simulink subsystem "control_law"  (R2023a)
settings: Solver=VariableStepAuto  StartTime=0.0  StopTime=10.0  RelTol=1e-3
values from neighbouring files (symbols this model uses):
  Kp_x = K(:,3:5)    [LQR_PI.m]    (also in full_loop.m = K(:,nref+1:np+nref); inner_loop.m = K(:,4:9))
undefined symbols (not defined in the file or in its folder): Kp_p, Kp_pitch, Kp_q, Kp_r, Kp_roll, Kp_vx, Kp_vy, Kp_vz, Kp_y, Kp_yaw, Kp_z, param, sat_p, sat_pitch, sat_q, sat_r, sat_roll, sat_Vx, sat_Vy, sat_Vz, sat_yaw, Td, Td_pos, Ti, Ti_pos
libraries: slpidlib x4, dspfdesign x3
settings Model: Creator=timme  LastModifiedBy=timme

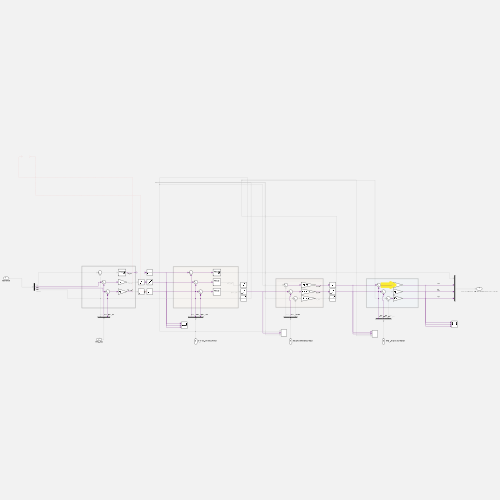
[thumbnail: Simulink's stored preview of the top-level diagram]
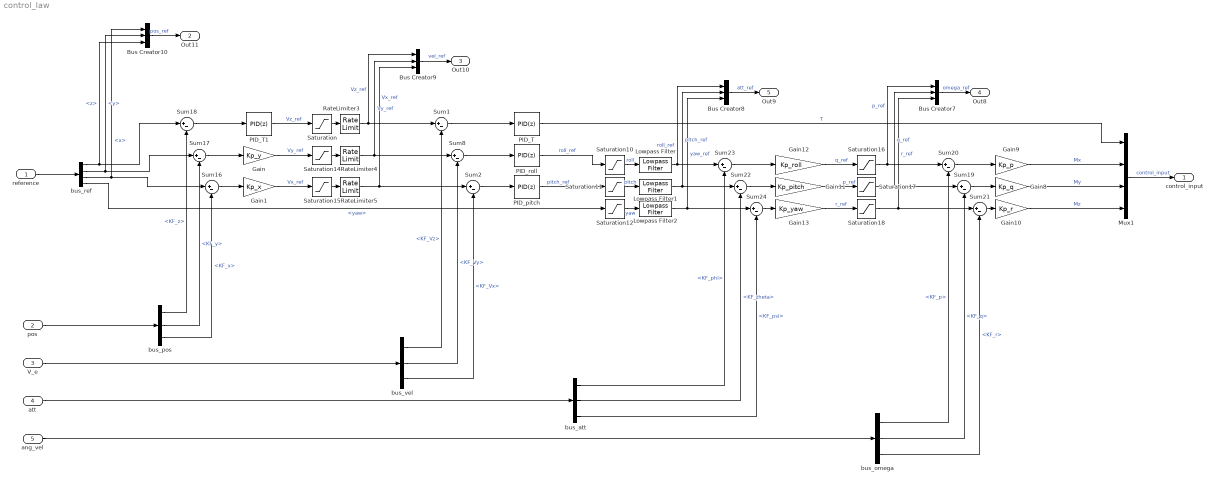
== system control_law ==
  reference : Inport
  pos : Inport  Port=2  Unit=m
  V_e : Inport  Port=3  Unit=m/s
  att : Inport  Port=4  Unit=rad
  ang_vel : Inport  Port=5  Unit=rad/s
  Bus Creator{7..10} (4 alike) : BusCreator  Inputs=3
  Gain : Gain  Gain=Kp_y
  Gain1 : Gain  Gain=Kp_x
  Gain10 : Gain  Gain=Kp_r
  Gain11 : Gain  Gain=Kp_pitch
  Gain12 : Gain  Gain=Kp_roll
  Gain13 : Gain  Gain=Kp_yaw
  Gain8 : Gain  Gain=Kp_q
  Gain9 : Gain  Gain=Kp_p
  Lowpass Filter : dspfdesign/Lowpass Filter  FilterType=IIR  DesignForMinimumOrder=on  FilterOrder=50  PassbandFrequency=1  StopbandFrequency=100  PassbandRipple=0.1  StopbandAttenuation=50  SampleRateMode=Specify on dialog  SampleRate=1000  SimulateUsing=Interpreted execution  roundingMode=Floor  coeffsDataTypeStr=fixdt(1,16)
  Lowpass Filter1 : dspfdesign/Lowpass Filter  FilterType=IIR  DesignForMinimumOrder=on  FilterOrder=50  PassbandFrequency=1  StopbandFrequency=100  PassbandRipple=0.1  StopbandAttenuation=50  SampleRateMode=Specify on dialog  SampleRate=1000  SimulateUsing=Interpreted execution  roundingMode=Floor  coeffsDataTypeStr=fixdt(1,16)
  Lowpass Filter2 : dspfdesign/Lowpass Filter  FilterType=IIR  DesignForMinimumOrder=on  FilterOrder=50  PassbandFrequency=1  StopbandFrequency=100  PassbandRipple=0.1  StopbandAttenuation=50  SampleRateMode=Specify on dialog  SampleRate=1000  SimulateUsing=Interpreted execution  roundingMode=Floor  coeffsDataTypeStr=fixdt(1,16)
  Mux1 : Mux
  PID_T : slpidlib/PID Controller  Controller=PID  Form=Parallel  TimeDomain=Discrete-time  UseExternalTs=off  SampleTime=param.dt  IntegratorMethod=Forward Euler  FilterMethod=Forward Euler  ControllerParametersSource=internal  P=Kp_vz  I=0  UseKiTs=on  D=0  N=100  UseFilter=on  TunerSelectOption=Transfer Function Based (PID Tuner App)  InitialConditionSource=internal  InitialConditionForIntegrator=0  InitialConditionForFilter=0  DifferentiatorICPrevScaledInput=0  ExternalReset=none  TrackingMode=off  Kt=1  LimitOutput=on  SatLimitsSource=internal  UpperSaturationLimit=2*param.m*param.g  LowerSaturationLimit=-2*param.m*param.g  LinearizeAsGain=on  AntiWindupMode=back-calculation  Kb=1  LimitIntegrator=off  UpperIntegratorSaturationLimit=inf  LowerIntegratorSaturationLimit=-inf  POutMin=[]  POutMax=[]  IOutMin=[]  IOutMax=[]  DOutMin=[]  DOutMax=[]  NOutMin=[]  NOutMax=[]  SumOutMin=[]  SumOutMax=[]  SaturationOutMin=[]  SaturationOutMax=[]  PParamMin=[]  PParamMax=[]  IParamMin=[]  IParamMax=[]  DParamMin=[]  DParamMax=[]  NParamMin=[]  NParamMax=[]  KbParamMin=[]  KbParamMax=[]  KtParamMin=[]  KtParamMax=[]  KbOutMin=[]  KbOutMax=[]  KtOutMin=[]  KtOutMax=[]  IntegratorOutMin=[]  IntegratorOutMax=[]  FilterOutMin=[]  FilterOutMax=[]  SumI1OutMin=[]  SumI1OutMax=[]  SumI2OutMin=[]  SumI2OutMax=[]  SumI3OutMin=[]  SumI3OutMax=[]  SumI4OutMin=[]  SumI4OutMax=[]  SumDOutMin=[]  SumDOutMax=[]  DifferentiatorOutMin=[]  DifferentiatorOutMax=[]  FilterDiffOutCoefMin=[]  FilterDiffOutCoefMax=[]  ReciprocalOutMin=[]  ReciprocalOutMax=[]  SumDenOutMin=[]  SumDenOutMax=[]  SumNumOutMin=[]  SumNumOutMax=[]  DivideOutMin=[]  DivideOutMax=[]  UdiffTsProdOutMin=[]  UdiffTsProdOutMax=[]  NTsProdOutMin=[]  NTsProdOutMax=[]  UintegralTsProdOutMin=[]  UintegralTsProdOutMax=[]  UngainTsProdOutMin=[]  UngainTsProdOutMax=[]  ClampingZeroOutDataTypeStr=Inherit: Inherit via back propagation  ClampingZeroOutMin=[]  ClampingZeroOutMax=[]  FilterDenConstantOutDataTypeStr=Inherit: Inherit via back propagation  FilterDenConstantOutMin=[]  FilterDenConstantOutMax=[]  PCopyOutDataTypeStr=Inherit: Inherit via back propagation  PCopyOutMin=[]  PCopyOutMax=[]  NCopyOutDataTypeStr=Inherit: Inherit via back propagation  NCopyOutMin=[]  NCopyOutMax=[]  IntegratorContinuousStateAttributes=''  IntegratorStateMustResolveToSignalObject=off  IntegratorRTWStateStorageClass=Auto  FilterContinuousStateAttributes=''  FilterStateMustResolveToSignalObject=off  FilterRTWStateStorageClass=Auto  ParallelPVariant=InternalParameters  IdealPVariant=Disabled  IVariant=InternalParameters  DVariant=InternalParameters  IntegratorVariant=Discrete  SatVariant=Enabled  AWVariant=BackCalculation  PCopyVariant=Disabled  TRVariant=Disabled  FdbkBlocksVariant=Forward  IdealPFdbkVariant=Disabled  SatFdbkVariant=Disabled  DerivativeFilterVariant=ForwardEulerFilter  NVariant=InternalParameters  NCopyVariant=Disabled  FilterICVariant=InternalICsFilter  IntegratorICVariant=InternalICs  ExternalResetVariant=Disabled  TRSumVariant=Passthrough  SumFdbkVariant=Disabled  SumVariant=Sum_PID  TsampFilterVariant=InternalTs  TsampNgainVariant=Passthrough  TsampIntegralVariant=Disabled_SignalSpec  ExternalSaturationOutDataTypeStr=Inherit: Same as second input
  PID_T1 : slpidlib/PID Controller  Controller=PID  Form=Parallel  TimeDomain=Discrete-time  UseExternalTs=off  SampleTime=param.dt  IntegratorMethod=Forward Euler  FilterMethod=Forward Euler  ControllerParametersSource=internal  P=Kp_z*(1+Td_pos/Ti_pos)  I=Kp_z/Ti_pos*param.dt  UseKiTs=on  D=Kp_z*Td_pos  N=100  UseFilter=on  TunerSelectOption=Transfer Function Based (PID Tuner App)  InitialConditionSource=internal  InitialConditionForIntegrator=0  InitialConditionForFilter=0  DifferentiatorICPrevScaledInput=0  ExternalReset=none  TrackingMode=off  Kt=1  LimitOutput=on  SatLimitsSource=internal  UpperSaturationLimit=sat_Vz  LowerSaturationLimit=-sat_Vz  LinearizeAsGain=on  AntiWindupMode=clamping  Kb=1  LimitIntegrator=off  UpperIntegratorSaturationLimit=inf  LowerIntegratorSaturationLimit=-inf  POutMin=[]  POutMax=[]  IOutMin=[]  IOutMax=[]  DOutMin=[]  DOutMax=[]  NOutMin=[]  NOutMax=[]  SumOutMin=[]  SumOutMax=[]  SaturationOutMin=[]  SaturationOutMax=[]  PParamMin=[]  PParamMax=[]  IParamMin=[]  IParamMax=[]  DParamMin=[]  DParamMax=[]  NParamMin=[]  NParamMax=[]  KbParamMin=[]  KbParamMax=[]  KtParamMin=[]  KtParamMax=[]  KbOutMin=[]  KbOutMax=[]  KtOutMin=[]  KtOutMax=[]  IntegratorOutMin=[]  IntegratorOutMax=[]  FilterOutMin=[]  FilterOutMax=[]  SumI1OutMin=[]  SumI1OutMax=[]  SumI2OutMin=[]  SumI2OutMax=[]  SumI3OutMin=[]  SumI3OutMax=[]  SumI4OutMin=[]  SumI4OutMax=[]  SumDOutMin=[]  SumDOutMax=[]  DifferentiatorOutMin=[]  DifferentiatorOutMax=[]  FilterDiffOutCoefMin=[]  FilterDiffOutCoefMax=[]  ReciprocalOutMin=[]  ReciprocalOutMax=[]  SumDenOutMin=[]  SumDenOutMax=[]  SumNumOutMin=[]  SumNumOutMax=[]  DivideOutMin=[]  DivideOutMax=[]  UdiffTsProdOutMin=[]  UdiffTsProdOutMax=[]  NTsProdOutMin=[]  NTsProdOutMax=[]  UintegralTsProdOutMin=[]  UintegralTsProdOutMax=[]  UngainTsProdOutMin=[]  UngainTsProdOutMax=[]  ClampingZeroOutDataTypeStr=Inherit: Inherit via back propagation  ClampingZeroOutMin=[]  ClampingZeroOutMax=[]  FilterDenConstantOutDataTypeStr=Inherit: Inherit via back propagation  FilterDenConstantOutMin=[]  FilterDenConstantOutMax=[]  PCopyOutDataTypeStr=Inherit: Inherit via back propagation  PCopyOutMin=[]  PCopyOutMax=[]  NCopyOutDataTypeStr=Inherit: Inherit via back propagation  NCopyOutMin=[]  NCopyOutMax=[]  IntegratorContinuousStateAttributes=''  IntegratorStateMustResolveToSignalObject=off  IntegratorRTWStateStorageClass=Auto  FilterContinuousStateAttributes=''  FilterStateMustResolveToSignalObject=off  FilterRTWStateStorageClass=Auto  ParallelPVariant=InternalParameters  IdealPVariant=Disabled  IVariant=InternalParameters  DVariant=InternalParameters  IntegratorVariant=Discrete  SatVariant=Enabled  AWVariant=DiscClampingParallel  PCopyVariant=Disabled  TRVariant=Disabled  FdbkBlocksVariant=Forward  IdealPFdbkVariant=Disabled  SatFdbkVariant=Disabled  DerivativeFilterVariant=ForwardEulerFilter  NVariant=InternalParameters  NCopyVariant=Disabled  FilterICVariant=InternalICsFilter  IntegratorICVariant=InternalICs  ExternalResetVariant=Disabled  TRSumVariant=Passthrough  SumFdbkVariant=Disabled  SumVariant=Sum_PID  TsampFilterVariant=InternalTs  TsampNgainVariant=Passthrough  TsampIntegralVariant=Disabled_SignalSpec  ExternalSaturationOutDataTypeStr=Inherit: Same as second input
  PID_pitch : slpidlib/PID Controller  Controller=PID  Form=Parallel  TimeDomain=Discrete-time  UseExternalTs=off  SampleTime=param.dt  IntegratorMethod=Forward Euler  FilterMethod=Forward Euler  ControllerParametersSource=internal  P=Kp_vx*(1+Td/Ti)  I=Kp_vx/Ti*param.dt  UseKiTs=on  D=Kp_vx*Td  N=100  UseFilter=on  TunerSelectOption=Transfer Function Based (PID Tuner App)  InitialConditionSource=internal  InitialConditionForIntegrator=0  InitialConditionForFilter=0  DifferentiatorICPrevScaledInput=0  ExternalReset=none  TrackingMode=off  Kt=1  LimitOutput=off  SatLimitsSource=internal  UpperSaturationLimit=inf  LowerSaturationLimit=-inf  LinearizeAsGain=on  AntiWindupMode=none  Kb=1  LimitIntegrator=off  UpperIntegratorSaturationLimit=inf  LowerIntegratorSaturationLimit=-inf  POutMin=[]  POutMax=[]  IOutMin=[]  IOutMax=[]  DOutMin=[]  DOutMax=[]  NOutMin=[]  NOutMax=[]  SumOutMin=[]  SumOutMax=[]  SaturationOutMin=[]  SaturationOutMax=[]  PParamMin=[]  PParamMax=[]  IParamMin=[]  IParamMax=[]  DParamMin=[]  DParamMax=[]  NParamMin=[]  NParamMax=[]  KbParamMin=[]  KbParamMax=[]  KtParamMin=[]  KtParamMax=[]  KbOutMin=[]  KbOutMax=[]  KtOutMin=[]  KtOutMax=[]  IntegratorOutMin=[]  IntegratorOutMax=[]  FilterOutMin=[]  FilterOutMax=[]  SumI1OutMin=[]  SumI1OutMax=[]  SumI2OutMin=[]  SumI2OutMax=[]  SumI3OutMin=[]  SumI3OutMax=[]  SumI4OutMin=[]  SumI4OutMax=[]  SumDOutMin=[]  SumDOutMax=[]  DifferentiatorOutMin=[]  DifferentiatorOutMax=[]  FilterDiffOutCoefMin=[]  FilterDiffOutCoefMax=[]  ReciprocalOutMin=[]  ReciprocalOutMax=[]  SumDenOutMin=[]  SumDenOutMax=[]  SumNumOutMin=[]  SumNumOutMax=[]  DivideOutMin=[]  DivideOutMax=[]  UdiffTsProdOutMin=[]  UdiffTsProdOutMax=[]  NTsProdOutMin=[]  NTsProdOutMax=[]  UintegralTsProdOutMin=[]  UintegralTsProdOutMax=[]  UngainTsProdOutMin=[]  UngainTsProdOutMax=[]  ClampingZeroOutDataTypeStr=Inherit: Inherit via back propagation  ClampingZeroOutMin=[]  ClampingZeroOutMax=[]  FilterDenConstantOutDataTypeStr=Inherit: Inherit via back propagation  FilterDenConstantOutMin=[]  FilterDenConstantOutMax=[]  PCopyOutDataTypeStr=Inherit: Inherit via back propagation  PCopyOutMin=[]  PCopyOutMax=[]  NCopyOutDataTypeStr=Inherit: Inherit via back propagation  NCopyOutMin=[]  NCopyOutMax=[]  IntegratorContinuousStateAttributes=''  IntegratorStateMustResolveToSignalObject=off  IntegratorRTWStateStorageClass=Auto  FilterContinuousStateAttributes=''  FilterStateMustResolveToSignalObject=off  FilterRTWStateStorageClass=Auto  ParallelPVariant=InternalParameters  IdealPVariant=Disabled  IVariant=InternalParameters  DVariant=InternalParameters  IntegratorVariant=Discrete  SatVariant=Disabled  AWVariant=Passthrough  PCopyVariant=Disabled  TRVariant=Disabled  FdbkBlocksVariant=Forward  IdealPFdbkVariant=Disabled  SatFdbkVariant=Disabled  DerivativeFilterVariant=ForwardEulerFilter  NVariant=InternalParameters  NCopyVariant=Disabled  FilterICVariant=InternalICsFilter  IntegratorICVariant=InternalICs  ExternalResetVariant=Disabled  TRSumVariant=Passthrough  SumFdbkVariant=Disabled  SumVariant=Sum_PID  TsampFilterVariant=InternalTs  TsampNgainVariant=Passthrough  TsampIntegralVariant=Disabled_SignalSpec  ExternalSaturationOutDataTypeStr=Inherit: Same as second input
  PID_roll : slpidlib/PID Controller  Controller=PID  Form=Parallel  TimeDomain=Discrete-time  UseExternalTs=off  SampleTime=param.dt  IntegratorMethod=Forward Euler  FilterMethod=Forward Euler  ControllerParametersSource=internal  P=Kp_vy*(1+Td/Ti)  I=Kp_vy/Ti*param.dt  UseKiTs=on  D=Kp_vy*Td  N=100  UseFilter=on  TunerSelectOption=Transfer Function Based (PID Tuner App)  InitialConditionSource=internal  InitialConditionForIntegrator=0  InitialConditionForFilter=0  DifferentiatorICPrevScaledInput=0  ExternalReset=none  TrackingMode=off  Kt=1  LimitOutput=off  SatLimitsSource=internal  UpperSaturationLimit=inf  LowerSaturationLimit=-inf  LinearizeAsGain=on  AntiWindupMode=none  Kb=1  LimitIntegrator=off  UpperIntegratorSaturationLimit=inf  LowerIntegratorSaturationLimit=-inf  POutMin=[]  POutMax=[]  IOutMin=[]  IOutMax=[]  DOutMin=[]  DOutMax=[]  NOutMin=[]  NOutMax=[]  SumOutMin=[]  SumOutMax=[]  SaturationOutMin=[]  SaturationOutMax=[]  PParamMin=[]  PParamMax=[]  IParamMin=[]  IParamMax=[]  DParamMin=[]  DParamMax=[]  NParamMin=[]  NParamMax=[]  KbParamMin=[]  KbParamMax=[]  KtParamMin=[]  KtParamMax=[]  KbOutMin=[]  KbOutMax=[]  KtOutMin=[]  KtOutMax=[]  IntegratorOutMin=[]  IntegratorOutMax=[]  FilterOutMin=[]  FilterOutMax=[]  SumI1OutMin=[]  SumI1OutMax=[]  SumI2OutMin=[]  SumI2OutMax=[]  SumI3OutMin=[]  SumI3OutMax=[]  SumI4OutMin=[]  SumI4OutMax=[]  SumDOutMin=[]  SumDOutMax=[]  DifferentiatorOutMin=[]  DifferentiatorOutMax=[]  FilterDiffOutCoefMin=[]  FilterDiffOutCoefMax=[]  ReciprocalOutMin=[]  ReciprocalOutMax=[]  SumDenOutMin=[]  SumDenOutMax=[]  SumNumOutMin=[]  SumNumOutMax=[]  DivideOutMin=[]  DivideOutMax=[]  UdiffTsProdOutMin=[]  UdiffTsProdOutMax=[]  NTsProdOutMin=[]  NTsProdOutMax=[]  UintegralTsProdOutMin=[]  UintegralTsProdOutMax=[]  UngainTsProdOutMin=[]  UngainTsProdOutMax=[]  ClampingZeroOutDataTypeStr=Inherit: Inherit via back propagation  ClampingZeroOutMin=[]  ClampingZeroOutMax=[]  FilterDenConstantOutDataTypeStr=Inherit: Inherit via back propagation  FilterDenConstantOutMin=[]  FilterDenConstantOutMax=[]  PCopyOutDataTypeStr=Inherit: Inherit via back propagation  PCopyOutMin=[]  PCopyOutMax=[]  NCopyOutDataTypeStr=Inherit: Inherit via back propagation  NCopyOutMin=[]  NCopyOutMax=[]  IntegratorContinuousStateAttributes=''  IntegratorStateMustResolveToSignalObject=off  IntegratorRTWStateStorageClass=Auto  FilterContinuousStateAttributes=''  FilterStateMustResolveToSignalObject=off  FilterRTWStateStorageClass=Auto  ParallelPVariant=InternalParameters  IdealPVariant=Disabled  IVariant=InternalParameters  DVariant=InternalParameters  IntegratorVariant=Discrete  SatVariant=Disabled  AWVariant=Passthrough  PCopyVariant=Disabled  TRVariant=Disabled  FdbkBlocksVariant=Forward  IdealPFdbkVariant=Disabled  SatFdbkVariant=Disabled  DerivativeFilterVariant=ForwardEulerFilter  NVariant=InternalParameters  NCopyVariant=Disabled  FilterICVariant=InternalICsFilter  IntegratorICVariant=InternalICs  ExternalResetVariant=Disabled  TRSumVariant=Passthrough  SumFdbkVariant=Disabled  SumVariant=Sum_PID  TsampFilterVariant=InternalTs  TsampNgainVariant=Passthrough  TsampIntegralVariant=Disabled_SignalSpec  ExternalSaturationOutDataTypeStr=Inherit: Same as second input
  RateLimiter3 : RateLimiter  RisingSlewLimit=2  FallingSlewLimit=-2  SampleTimeMode=inherited
  RateLimiter4 : RateLimiter  RisingSlewLimit=2  FallingSlewLimit=-2  SampleTimeMode=inherited
  RateLimiter5 : RateLimiter  RisingSlewLimit=2  FallingSlewLimit=-2  SampleTimeMode=inherited
  Saturation : Saturate  UpperLimit=sat_Vz  LowerLimit=-sat_Vz
  Saturation10 : Saturate  UpperLimit=sat_roll*pi/180  LowerLimit=-sat_roll*pi/180
  Saturation11 : Saturate  UpperLimit=sat_pitch*pi/180  LowerLimit=-sat_pitch*pi/180
  Saturation12 : Saturate  UpperLimit=sat_yaw*pi/180  LowerLimit=-sat_yaw*pi/180
  Saturation14 : Saturate  UpperLimit=sat_Vy  LowerLimit=-sat_Vy
  Saturation15 : Saturate  UpperLimit=sat_Vx  LowerLimit=-sat_Vx
  Saturation16 : Saturate  UpperLimit=sat_p*pi/180  LowerLimit=-sat_p*pi/180
  Saturation17 : Saturate  UpperLimit=sat_q*pi/180  LowerLimit=-sat_q*pi/180
  Saturation18 : Saturate  UpperLimit=sat_r*pi/180  LowerLimit=-sat_r*pi/180
  Sum{1..2,8,16..24} (12 alike) : Sum  Inputs=|+-
  bus_att : BusSelector  OutputSignals=KF_phi,KF_theta,KF_psi
  bus_omega : BusSelector  OutputSignals=KF_p,KF_q,KF_r
  bus_pos : BusSelector  OutputSignals=KF_z,KF_y,KF_x
  bus_ref : BusSelector  OutputSignals=z,y,x,yaw
  bus_vel : BusSelector  OutputSignals=KF_Vz,KF_Vy,KF_Vx
  control_input : Outport
  Out11 : Outport  Port=2
  Out10 : Outport  Port=3
  Out8 : Outport  Port=4
  Out9 : Outport  Port=5
  wires:
  PID_roll/1 -> Saturation10/1  "roll_ref"
  Sum24/1 -> Gain13/1
  bus_att/1 -> Sum23/2  "<KF_phi>"
  Mux1/1 -> control_input/1  "control_input"
  PID_pitch/1 -> Saturation11/1  "pitch_ref"
  Gain13/1 -> Saturation18/1  "r_ref"
  att/1 -> bus_att/1
  V_e/1 -> bus_vel/1
  Gain/1 -> Saturation14/1  "Vy_ref"
  Sum19/1 -> Gain8/1
  Gain1/1 -> Saturation15/1  "Vx_ref"
  Sum18/1 -> PID_T1/1
  bus_att/3 -> Sum24/2  "<KF_psi>"
  reference/1 -> bus_ref/1
  ang_vel/1 -> bus_omega/1
  Saturation15/1 -> RateLimiter5/1
  bus_pos/1 -> Sum18/2  "<KF_z>"
  pos/1 -> bus_pos/1
  bus_omega/3 -> Sum21/2  "<KF_r>"
  bus_ref/4 -> Saturation12/1  "<yaw>"
  PID_T/1 -> Mux1/1  "T"
  bus_omega/2 -> Sum19/2  "<KF_q>"
  bus_omega/1 -> Sum20/2  "<KF_p>"
  bus_att/2 -> Sum22/2  "<KF_theta>"
  bus_vel/1 -> Sum1/2  "<KF_Vz>"
  bus_vel/3 -> Sum2/2  "<KF_Vx>"
  bus_vel/2 -> Sum8/2  "<KF_Vy>"
  bus_pos/3 -> Sum16/2  "<KF_x>"
  bus_pos/2 -> Sum17/2  "<KF_y>"
  Gain10/1 -> Mux1/4  "Mz"
  Gain11/1 -> Saturation17/1  "p_ref"
  Gain12/1 -> Saturation16/1  "q_ref"
  Gain8/1 -> Mux1/3  "My"
  Gain9/1 -> Mux1/2  "Mx"
  PID_T1/1 -> Saturation/1  "Vz_ref"
  Saturation14/1 -> RateLimiter4/1
  Sum16/1 -> Gain1/1
  Sum17/1 -> Gain/1
  Sum1/1 -> PID_T/1
  Sum20/1 -> Gain9/1
  Sum21/1 -> Gain10/1
  Sum22/1 -> Gain11/1
  Sum23/1 -> Gain12/1
  Sum2/1 -> PID_pitch/1
  Sum8/1 -> PID_roll/1
  Saturation/1 -> RateLimiter3/1
  Saturation12/1 -> Lowpass Filter2/1  "yaw"
  Saturation10/1 -> Lowpass Filter/1  "roll"
  Saturation11/1 -> Lowpass Filter1/1  "pitch"
  bus_ref/2 -> Sum17/1, Bus Creator10/2  "<y>"
  bus_ref/1 -> Sum18/1, Bus Creator10/3  "<z>"
  bus_ref/3 -> Sum16/1, Bus Creator10/1  "<x>"
  Bus Creator10/1 -> Out11/1  "pos_ref"
  RateLimiter4/1 -> Sum8/1, Bus Creator9/2  "Vy_ref"
  RateLimiter3/1 -> Sum1/1, Bus Creator9/1  "Vz_ref"
  RateLimiter5/1 -> Sum2/1, Bus Creator9/3  "Vx_ref"
  Bus Creator9/1 -> Out10/1  "vel_ref"
  Saturation16/1 -> Sum20/1, Bus Creator7/1  "p_ref"
  Bus Creator8/1 -> Out9/1  "att_ref"
  Bus Creator7/1 -> Out8/1  "omega_ref"
  Lowpass Filter/1 -> Bus Creator8/1, Sum23/1  "roll_ref"
  Lowpass Filter2/1 -> Bus Creator8/3, Sum24/1  "yaw_ref"
  Saturation17/1 -> Sum19/1, Bus Creator7/2  "q_ref"
  Lowpass Filter1/1 -> Bus Creator8/2, Sum22/1  "pitch_ref"
  Saturation18/1 -> Sum21/1, Bus Creator7/3  "r_ref"
